simulink model "Funcion_a_trozos"  (R2023a)
settings: Solver=VariableStepAuto  StartTime=0.0  StopTime=10.0  RelTol=1e-3
settings Model: Creator=Nacho Andrade  LastModifiedBy=Nacho Andrade

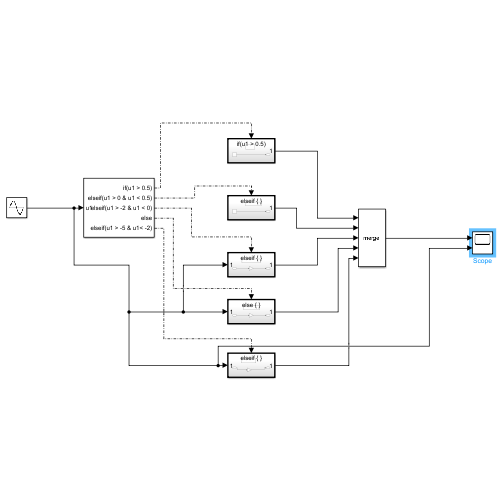
[thumbnail: Simulink's stored preview of the top-level diagram]
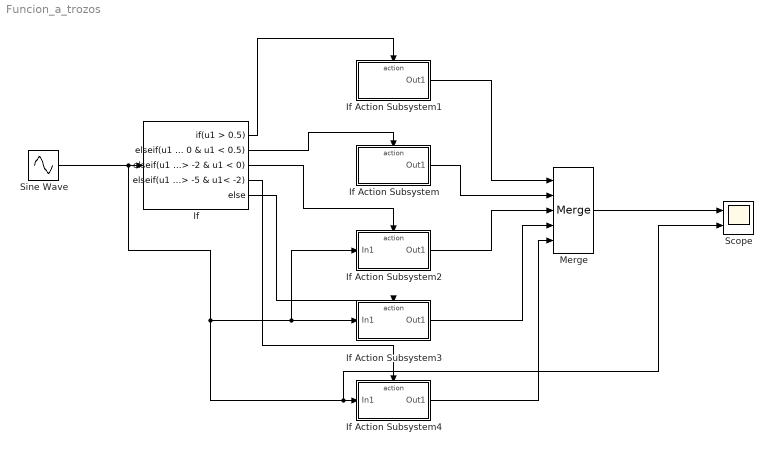
== system Funcion_a_trozos ==
  If : If  IfExpression=u1 > 0.5  ElseIfExpressions=u1 > 0 & u1 < 0.5,u1 > -2 & u1 < 0,u1 > -5 & u1< -2  ZeroCross=off
  If Action Subsystem : Subsystem  TreatAsAtomicUnit=on
  If Action Subsystem1 : Subsystem  TreatAsAtomicUnit=on
  If Action Subsystem2 : Subsystem  TreatAsAtomicUnit=on
  If Action Subsystem3 : Subsystem  TreatAsAtomicUnit=on
  If Action Subsystem4 : Subsystem  TreatAsAtomicUnit=on
  Merge : Merge  Inputs=5
  Scope : Scope  NumInputPorts=2
  Sine Wave : Sin  Amplitude=6  SampleTime=0
  wires:
  If/1 -> If Action Subsystem1/Action
  If/2 -> If Action Subsystem/Action
  If/3 -> If Action Subsystem2/Action
  If/5 -> If Action Subsystem3/Action
  If/4 -> If Action Subsystem4/Action
  Sine Wave/1 -> Scope/2, If Action Subsystem4/1(In1), If Action Subsystem2/1(In1), If Action Subsystem3/1(In1), If/1
  If Action Subsystem1/1(Out1) -> Merge/1
  If Action Subsystem/1(Out1) -> Merge/2
  If Action Subsystem2/1(Out1) -> Merge/3
  If Action Subsystem3/1(Out1) -> Merge/4
  If Action Subsystem4/1(Out1) -> Merge/5
  Merge/1 -> Scope/1

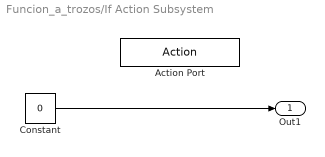
== system Funcion_a_trozos/If Action Subsystem ==
  Action Port : ActionPort  ActionPortLabel=elseif(u1 > 0 & u1 < 0.5)
  Constant : Constant  Value=0
  Out1 : Outport
  wires:
  Constant/1 -> Out1/1

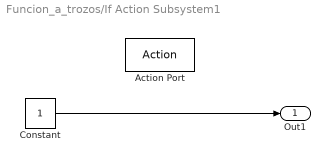
== system Funcion_a_trozos/If Action Subsystem1 ==
  Action Port : ActionPort  ActionPortLabel=if(u1 > 0.5)
  Constant : Constant
  Out1 : Outport
  wires:
  Constant/1 -> Out1/1

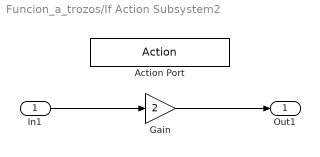
== system Funcion_a_trozos/If Action Subsystem2 ==
  In1 : Inport
  Action Port : ActionPort  ActionPortLabel=elseif(u1 > -2 & u1 < 0)
  Gain : Gain  Gain=2
  Out1 : Outport
  wires:
  In1/1 -> Gain/1
  Gain/1 -> Out1/1

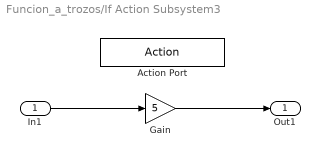
== system Funcion_a_trozos/If Action Subsystem3 ==
  In1 : Inport
  Action Port : ActionPort  ActionPortLabel=else
  Gain : Gain  Gain=5
  Out1 : Outport
  wires:
  In1/1 -> Gain/1
  Gain/1 -> Out1/1

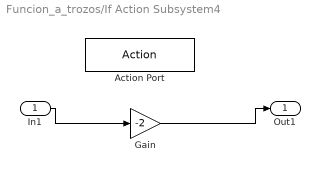
== system Funcion_a_trozos/If Action Subsystem4 ==
  In1 : Inport
  Action Port : ActionPort  ActionPortLabel=elseif(u1 > -5 & u1< -2)
  Gain : Gain  Gain=-2
  Out1 : Outport
  wires:
  In1/1 -> Gain/1
  Gain/1 -> Out1/1
